simulink library "CapellaElements"  (R2018a)
settings: Solver=VariableStepAuto  StartTime=0.0  StopTime=10.0  RelTol=1e-3
settings Model: Creator=XXXX  LastModifiedBy=XXXX
settings DataIOCC: ReturnWorkspaceOutputs=on
settings SFSimCC: SimUseLocalCustomCode=on
settings RTWCC: RTWUseLocalCustomCode=on

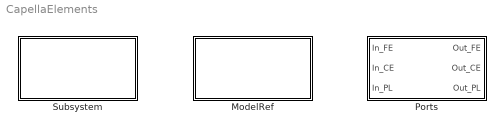
== system CapellaElements ==
  ModelRef : Subsystem
  Ports : Subsystem
  Subsystem : Subsystem

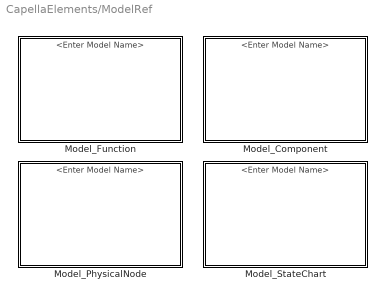
== system CapellaElements/ModelRef ==
  Model_Component : ModelReference  SimulationMode=Normal
      settings: CopyFcn=set_param(gcbh,'LinkStatus','none');
      mask Display:
      | image('Capella_logo.png', [2, 2, 20, 20*97/123])
      | color('darkBlue'); disp('{\itComponent}', 'texmode', 'on')
  Model_Function : ModelReference  SimulationMode=Normal
      settings: CopyFcn=set_param(gcbh,'LinkStatus','none');
      mask Display:
      | image('Capella_logo.png', [2, 2, 20, 20*97/123])
      | color('darkGreen');disp('Function')
  Model_PhysicalNode : ModelReference  SimulationMode=Normal
      settings: CopyFcn=set_param(gcbh,'LinkStatus','none');
      mask Display:
      | image('Capella_logo.png', [2, 2, 20, 20*97/123])
      | color('black'); disp('Physical Node');
  Model_StateChart : ModelReference  SimulationMode=Normal
      settings: CopyFcn=set_param(gcbh,'LinkStatus','none');
      mask Display:
      | image('Capella_logo.png', [2, 2, 20, 20*97/123])
      | color('black');disp('M&S')

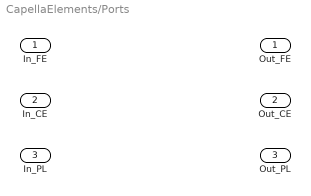
== system CapellaElements/Ports ==
  In_FE : Inport
      settings: CopyFcn=set_param(gcbh,'LinkStatus','none');
  In_CE : Inport  Port=2
      settings: CopyFcn=set_param(gcbh,'LinkStatus','none');
  In_PL : Inport  Port=3
      settings: CopyFcn=set_param(gcbh,'LinkStatus','none');
  Out_FE : Outport
      settings: CopyFcn=set_param(gcbh,'LinkStatus','none');
  Out_CE : Outport  Port=2
      settings: CopyFcn=set_param(gcbh,'LinkStatus','none');
  Out_PL : Outport  Port=3
      settings: CopyFcn=set_param(gcbh,'LinkStatus','none');

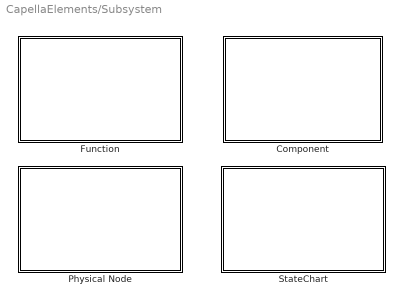
== system CapellaElements/Subsystem ==
  Component : Subsystem
      settings: CopyFcn=set_param(gcbh,'LinkStatus','none');
      mask Display:
      | image('Capella_logo.png', [2, 2, 20, 20*97/123])
      | color('darkBlue'); disp('{\itComponent}', 'texmode', 'on')
  Function : Subsystem
      settings: CopyFcn=set_param(gcbh,'LinkStatus','none');
      mask Display:
      | image('Capella_logo.png', [2, 2, 20, 20*97/123])
      | color('darkGreen');disp('Function')
  Physical Node : Subsystem
      settings: CopyFcn=set_param(gcbh,'LinkStatus','none');
      mask Display:
      | image('Capella_logo.png', [2, 2, 20, 20*97/123])
      | color('black'); disp('Physical Node');
  StateChart : Stateflow chart  TreatAsAtomicUnit=on
      settings: CopyFcn=set_param(gcbh,'LinkStatus','none');

== system CapellaElements/Subsystem/Component ==

== system CapellaElements/Subsystem/Function ==

== system CapellaElements/Subsystem/Physical Node ==

== stateflow chart CapellaElements/Subsystem/StateChart ==
